simulink model "Ex_6"  (R2020a)
settings: Solver=VariableStepAuto  StartTime=0.0  StopTime=10.0  RelTol=1e-6
values from neighbouring files (symbols this model uses):
  B = 0.0025    [m6.m]    (also in m7.m)
  J = 0.02365    [m6.m]    (also in m7.m)
  La = 0.12    [m6.m]    (also in m7.m)
  Lase = 0.0018    [m6.m]
  Lash = 1.8    [m6.m]
  Lse = 0.012    [m6.m]
  Lsh = 0.03    [m6.m]
  Lshse = 0.001    [m6.m]
  Ra = 1.50    (= 1.5)    [m6.m]    (also in m7.m)
  Rse = 0.7    [m6.m]
  Rsh = 270    [m6.m]
  Vdc = 230    [m6.m]
settings Model: Creator=VAISHNAVI LOPAMUDRA  LastModifiedBy=abhin

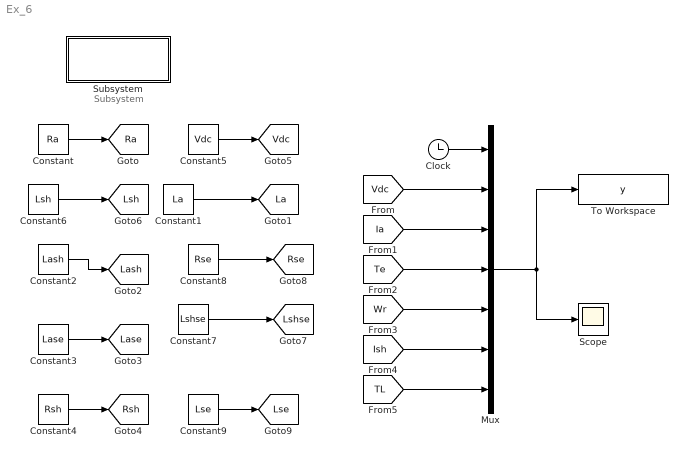
== system Ex_6 ==
  note: Subsystem
  Clock : Clock
  Constant : Constant  Value=Ra
  Constant1 : Constant  Value=La
  Constant2 : Constant  Value=Lash
  Constant3 : Constant  Value=Lase
  Constant4 : Constant  Value=Rsh
  Constant5 : Constant  Value=Vdc
  Constant6 : Constant  Value=Lsh
  Constant7 : Constant  Value=Lshse
  Constant8 : Constant  Value=Rse
  Constant9 : Constant  Value=Lse
  Mux : Mux  Inputs=7
  Scope : Scope
  Subsystem : Subsystem
  To Workspace : ToWorkspace  VariableName=y  SampleTime=-1
  tag scope: La=global, Lase=global, Lash=global, Lse=global, Lsh=global, Lshse=global, Ra=global, Rse=global, Rsh=global, Vdc=global
  wires:
  Constant2/1 -> [Lash]
  Constant3/1 -> [Lase]
  Constant4/1 -> [Rsh]
  Constant/1 -> [Ra]
  Constant1/1 -> [La]
  Constant5/1 -> [Vdc]
  Constant6/1 -> [Lsh]
  Constant7/1 -> [Lshse]
  Constant8/1 -> [Rse]
  Constant9/1 -> [Lse]
  [TL] -> Mux/7
  [Ish] -> Mux/6
  [Wr] -> Mux/5
  [Te] -> Mux/4
  [Ia] -> Mux/3
  [Vdc] -> Mux/2
  Clock/1 -> Mux/1
  Mux/1 -> To Workspace/1, Scope/1

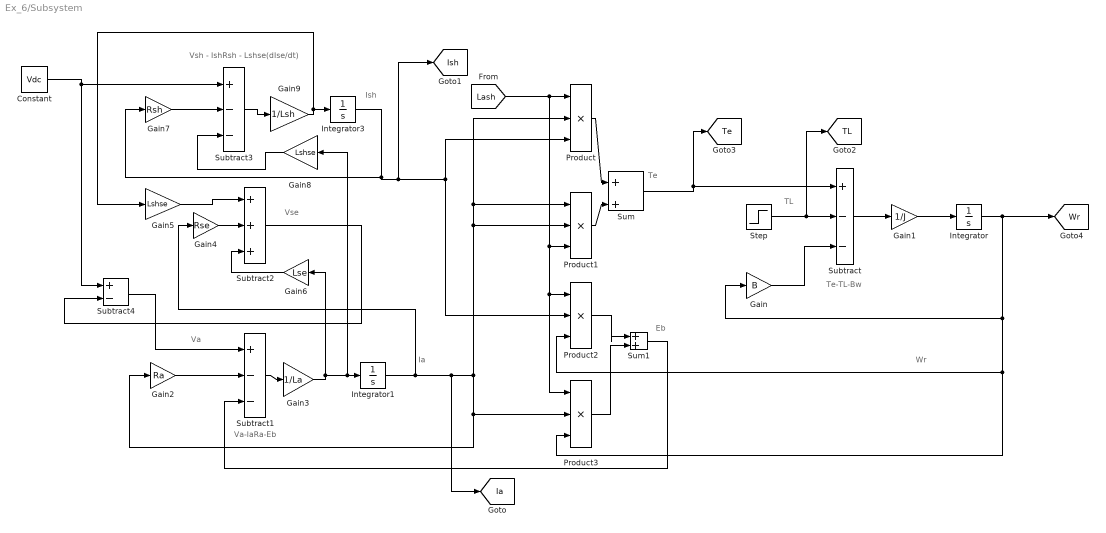
== system Ex_6/Subsystem ==
  note: Vsh - IshRsh - Lshse(dIse/dt)
  note: Vse
  note: Va
  note: Va-IaRa-Eb
  note: Te-TL-Bw
  note: Ish
  note: TL
  note: Te
  note: Wr
  note: Eb
  note: Ia
  Constant : Constant  Value=Vdc
  Gain : Gain  Gain=B
  Gain1 : Gain  Gain=1/J
  Gain2 : Gain  Gain=Ra
  Gain3 : Gain  Gain=1/La
  Gain4 : Gain  Gain=Rse
  Gain5 : Gain  Gain=Lshse
  Gain6 : Gain  Gain=Lse
  Gain7 : Gain  Gain=Rsh
  Gain8 : Gain  Gain=Lshse
  Gain9 : Gain  Gain=1/Lsh
  Integrator : Integrator
  Integrator1 : Integrator
  Integrator3 : Integrator
  Product{,1..3} (4 alike) : Product  Inputs=3
  Step : Step  Time=3  After=10  SampleTime=0
  Subtract : Sum  Inputs=+--
  Subtract1 : Sum  Inputs=+--
  Subtract2 : Sum  Inputs=+++
  Subtract3 : Sum  Inputs=+--
  Subtract4 : Sum  Inputs=+-
  Sum : Sum  Inputs=|++
  Sum1 : Sum  Inputs=|++
  tag scope: Ia=global, Ish=global, TL=global, Te=global, Wr=global
  wires:
  Step/1 -> [TL], Subtract/2
  Gain/1 -> Subtract/3
  Subtract/1 -> Gain1/1
  Gain1/1 -> Integrator/1
  Integrator/1 -> [Wr], Product3/3, Product2/3, Gain/1
  Product/1 -> Sum/1
  Product1/1 -> Sum/2
  Sum/1 -> [Te], Subtract/1
  [Lash] -> Product3/1, Product2/1, Product1/3, Product/1
  Product2/1 -> Sum1/1
  Product3/1 -> Sum1/2
  Sum1/1 -> Subtract1/3
  Gain2/1 -> Subtract1/2
  Subtract1/1 -> Gain3/1
  Integrator1/1 -> [Ia], Product1/2, Product1/1, Product/2, Gain2/1, Product3/2, Gain4/1
  Gain4/1 -> Subtract2/2
  Gain6/1 -> Subtract2/3
  Constant/1 -> Subtract4/1, Subtract3/1
  Gain7/1 -> Subtract3/2
  Gain8/1 -> Subtract3/3
  Subtract3/1 -> Gain9/1
  Gain9/1 -> Gain5/1, Integrator3/1
  Gain5/1 -> Subtract2/1
  Subtract2/1 -> Subtract4/2
  Subtract4/1 -> Subtract1/1
  Integrator3/1 -> Gain7/1, Product/3, Product2/2, [Ish]
  Gain3/1 -> Gain6/1, Gain8/1, Integrator1/1
